simulink model "Es1_1slx"  (R2014a)
settings: Solver=ode45  StartTime=0.0  StopTime=30.0  RelTol=1e-3
libraries: cstblocks x2
settings Model: Creator=UTENTE  LastModifiedBy=UTENTE

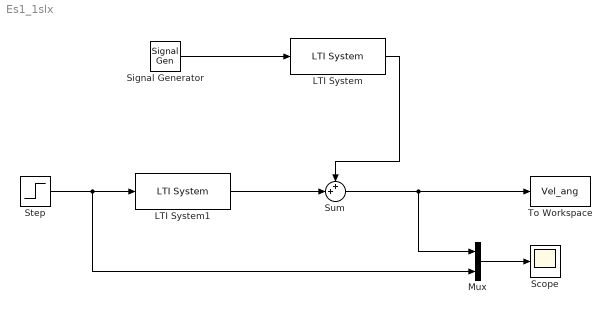
== system Es1_1slx ==
  LTI System : cstblocks/LTI System  sys=F2  IC=[]
  LTI System1 : cstblocks/LTI System  sys=F1  IC=[]
  Mux : Mux  Inputs=2
  Scope : Scope
  Signal Generator : SignalGenerator  WaveForm=square  Amplitude=0.05  Frequency=0.1
  Step : Step  Time=0  After=u  SampleTime=0
  Sum : Sum  Inputs=++|
  To Workspace : ToWorkspace  VariableName=Vel_ang  SaveFormat=Timeseries  SampleTime=-1
  wires:
  Signal Generator/1 -> LTI System/1
  LTI System/1 -> Sum/1
  Step/1 -> Mux/2, LTI System1/1
  LTI System1/1 -> Sum/2
  Sum/1 -> Mux/1, To Workspace/1
  Mux/1 -> Scope/1
